simulink model "DSBSC_SIM"  (R2024a)
settings: Solver=VariableStepAuto  StartTime=0.0  StopTime=10.0  RelTol=1e-3
libraries: dspfdesign x1
settings Model: Creator=vnrvjiet  LastModifiedBy=adity
settings SolverCC: AlgebraicLoopSolver=TrustRegion
settings DataIOCC: ReturnWorkspaceOutputs=off
settings DebuggingCC: UnconnectedInputMsg=warning  UnconnectedOutputMsg=warning  UnconnectedLineMsg=warning  ArithmeticOperatorsInVariantConditions=warning
settings ModelReferenceCC: EnableRefExpFcnMdlSchedulingChecks=on
settings SFSimCC: SimUseLocalCustomCode=off  CustomCodeUndefinedFunction=UseInterfaceOnly
settings RTWCC: RTWUseLocalCustomCode=off  GPUComputeCapability=3.5

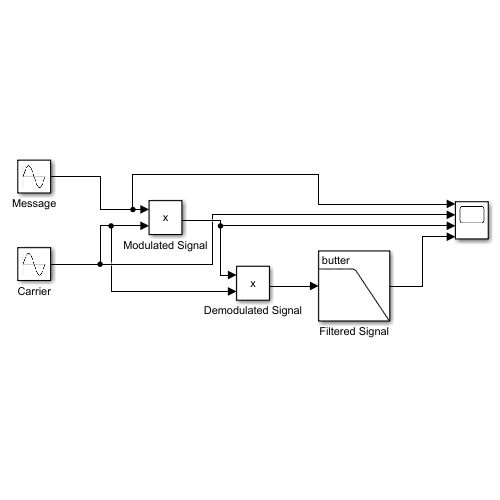
[thumbnail: Simulink's stored preview of the top-level diagram]
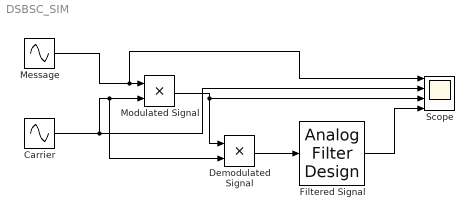
== system DSBSC_SIM ==
  Carrier : Sin  Amplitude=3  Frequency=2*pi*10  Phase=pi/2  SampleTime=0
  Demodulated Signal : Product
  Filtered Signal : dspfdesign/Analog Filter Design  method=Butterworth  filttype=Lowpass  N=8  Wlo=30  Whi=80  Rp=2  Rs=40
  Message : Sin  Amplitude=3  Frequency=2*pi*1  SampleTime=0
  Modulated Signal : Product
  Scope : Scope  NumInputPorts=4
  wires:
  Carrier/1 -> Scope/2, Demodulated Signal/2, Modulated Signal/2
  Message/1 -> Scope/1, Modulated Signal/1
  Modulated Signal/1 -> Scope/3, Demodulated Signal/1
  Demodulated Signal/1 -> Filtered Signal/1
  Filtered Signal/1 -> Scope/4
